simulink model "sys"  (R2021a)
settings: Solver=VariableStepAuto  StartTime=0.0  StopTime=10.0  RelTol=1e-3
settings Model: Creator=Suman  LastModifiedBy=Suman

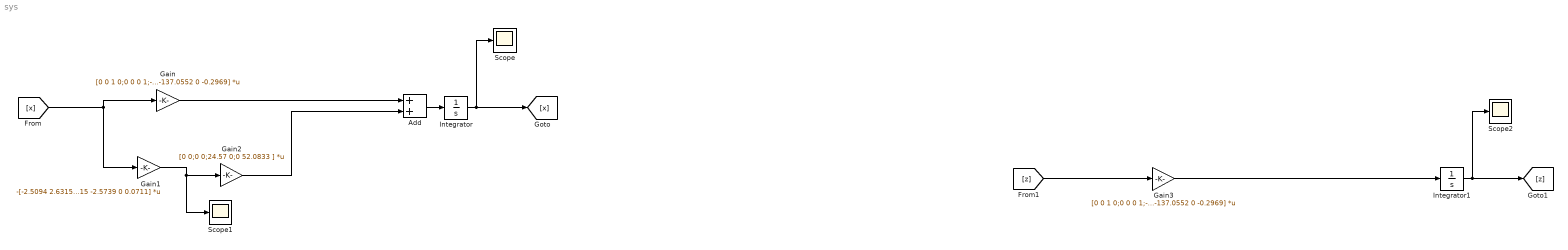
== system sys ==
  Add : Sum
  Gain : Gain  Gain=[0 0 1 0;0 0 0 1;-64.6551 64.6551 -0.1990 0;137.0552 -137.0552 0 -0.2969]  Multiplication=Matrix(K*u) (u vector)
  Gain1 : Gain  Gain=-[-2.5094 2.6315 0.1547 0;2.6315 -2.5739 0 0.0711]  Multiplication=Matrix(K*u) (u vector)
  Gain2 : Gain  Gain=[0 0;0 0;24.57 0;0 52.0833 ]  Multiplication=Matrix(K*u)
  Gain3 : Gain  Gain=[0 0 1 0;0 0 0 1;-64.6551 64.6551 -0.1990 0;137.0552 -137.0552 0 -0.2969]  Multiplication=Matrix(K*u) (u vector)
  Integrator : Integrator  InitialCondition=[0;2.75;1;1]
  Integrator1 : Integrator  InitialCondition=[0;2.75;1;1]
  Scope : Scope
  Scope1 : Scope
  Scope2 : Scope
  wires:
  [x] -> Gain1/1, Gain/1
  Gain/1 -> Add/1
  Gain2/1 -> Add/2
  Add/1 -> Integrator/1
  Integrator/1 -> Scope/1, [x]
  Gain1/1 -> Scope1/1, Gain2/1
  Integrator1/1 -> Scope2/1, [z]
  [z] -> Gain3/1
  Gain3/1 -> Integrator1/1
